simulink model "INS_Code_Simulink"  (R2023b)
settings: Solver=FixedStepAuto  StartTime=0.0  StopTime=60  FixedStep=0.01  RelTol=1e-3
settings Model: Creator=HP  LastModifiedBy=Ali
settings DebuggingCC: UnconnectedInputMsg=warning  UnconnectedOutputMsg=warning  UnconnectedLineMsg=warning
settings ModelReferenceCC: EnableRefExpFcnMdlSchedulingChecks=on
settings RTWCC: DLArmComputeVersion=19.05

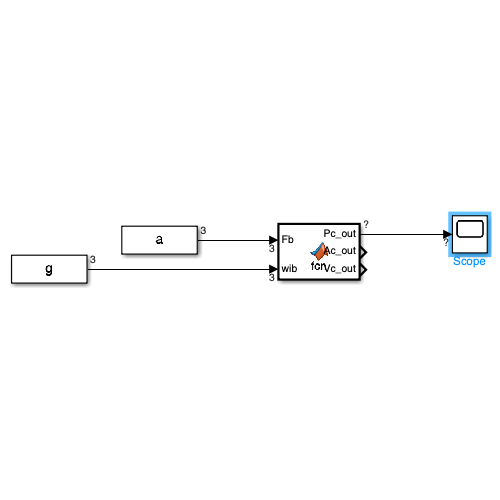
[thumbnail: Simulink's stored preview of the top-level diagram]
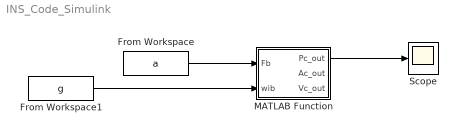
== system INS_Code_Simulink ==
  From Workspace : FromWorkspace  VariableName=a
  From Workspace1 : FromWorkspace  VariableName=g
  MATLAB Function : MATLAB Function  TreatAsAtomicUnit=on
  Scope : Scope
  wires:
  From Workspace/1 -> MATLAB Function/1(Fb)
  From Workspace1/1 -> MATLAB Function/2(wib)
  MATLAB Function/1(Pc_out) -> Scope/1

== matlab function INS_Code_Simulink/MATLAB Function ==
  data: Fb input; Pc_out output; wib input; Ac_out output; Vc_out output
function [Pc_out,Ac_out,Vc_out] = fcn(Fb,wib)

%%
persistent Pc Ac Vc Cbn
if isempty(Pc)
    Pc=[0;0;0];
end
if isempty(Ac)
    Ac=[0;0;0];
    Cbn=CalcCbn(Ac);
end
if isempty(Vc)
    Vc=[0;0;0];
end
%% parameters:
%% Sample rate
DeltaT = 0.01; %Sample time
%% Earth Parameters
f = 1/298.2572236;
e = 0.0818191908426;
R0 = 6378137;
ee = e*e;
Omega_e = 7.29211651452621e-5;
%% Sin and Cos Lateral
CCLA = cos(Pc(1,1));
SCLA = sin(Pc(1,1));
SC2LA = sin(2*Pc(1,1));
%% Calculating Ground Radious
RG = R0*(1-f*SCLA*SCLA); %Gussian Radius
RN = R0*(1-ee)/(1-ee*SCLA*SCLA)^1.5;
RE = R0/(1-ee*SCLA*SCLA)^0.5;
%% Sin and Cos Euler Angles
SCR = sin(Ac(1,1));
CCR = cos(Ac(1,1));
SCP = sin(Ac(2,1));
CCP = cos(Ac(2,1));
TCP = SCP/CCP;
%%%%%%%%%%%%%%%%%%%%%%%%%%%%%%%%%%%%%%%%%%%%%%%%%%%%%%%%%%%%%%%%%%%%%%%%%%%
%%%%%%%%%%%%%%%%%%%%%%%%%%%%%%%%%%%%%%%%%%%%%%%%%%%%%%%%%%%%%%%%%%%%%%%%%%%
%% Body rate at NED frame from body rate at inertial frame
win1 = Omega_e*CCLA + Vc(2,1)/(RE+Pc(3,1));
win2 = -1* Vc(1,1)/(RN+Pc(3,1));
win3 = -1*Omega_e*SCLA - Vc(2,1)*SCLA/((RE+Pc(3,1))*CCLA);
win=[win1;win2;win3];
%%
wnb = wib -Cbn'*win;
%% Calculating new attitude rate from body rate at NED
ADot1 = wnb(1,1)+(wnb(2,1)*SCR + wnb(3,1)*CCR)*TCP;
ADot2 = wnb(2,1)*CCR -wnb(3,1)*SCR;
ADot3 = (wnb(2,1)*SCR+ wnb(3,1)*CCR)/CCP;
ADot =[ADot1;ADot2;ADot3];
%% Calculating new attitude angles
Ac = Ac + ADot*DelatT;
%% Calculating Cos transfer Matrix for trasferring  from body frame to navigation frame
Cbn=CalcCbn(Ac);
%% Velocity Update
%% Transferring Force from body frame to NED frame
Fn=Cbn*Fb;
%% Calculating Gravity vector
gh0 = 9.780318*(1+5.3024e-3*SCLA*SCLA - 5.9e-6*SC2LA);
gh = gh0/(1+Pc(3,1)/RG)^2;
Gn1=0;
Gn2=0;
Gn3=gh;
Gn=[Gn1;Gn2;Gn3];
%% Calculating Vdot
VDot1 = Vc(1,1)*Vc(3,1)/(RN+Pc(3,1))-Vc(2,1)*Vc(2,1)*SCLA/((RE+Pc(3,1))*CCLA)...
           -2*Omega_e*Vc(2,1)*SCLA;
VDot2 = 2*Omega_e*Vc(1,1)*SCLA + Vc(1,1)*Vc(2,1)*SCLA/((RE+Pc(3,1))*CCLA)...
           +2*Omega_e*Vc(3,1)*CCLA + Vc(2,1)*Vc(3,1)/(RE+Pc(3,1));
VDot3 = -2*Omega_e*Vc(2,1)*CCLA - Vc(2,1)*Vc(2,1)/(RE+Pc(3,1))...
           -Vc(1,1)*Vc(1,1)/(RN+Pc(3,1));
VDot=[VDot1;VDot2;VDot3];
VDot = Fn+VDot+Gn;
%% Calculating new linear velocity:euler discrtization
Vc = Vc + VDot*DeltaT;
%% Position Update:
PDot1 = Vc(1,1)/(RN+Pc(3,1));
PDot2 = Vc(2,1)/((RE+Pc(3,1))*CCLA);
PDot3 = -1 * Vc(3,1);
PDot=[PDot1;PDot2;PDot3];
%% Calculating new geodetic position
Pc = Pc+PDot*DeltaT;
%% Outputs
Pc_out = Pc;
Vc_out = Vc;
Ac_out = Ac;
%%
